simulink model "Punto_5"  (R2024b)
settings: Solver=VariableStepAuto  StartTime=0.0  StopTime=2  RelTol=1e-3
settings Model: Creator=Andres Felipe  LastModifiedBy=Andres Felipe

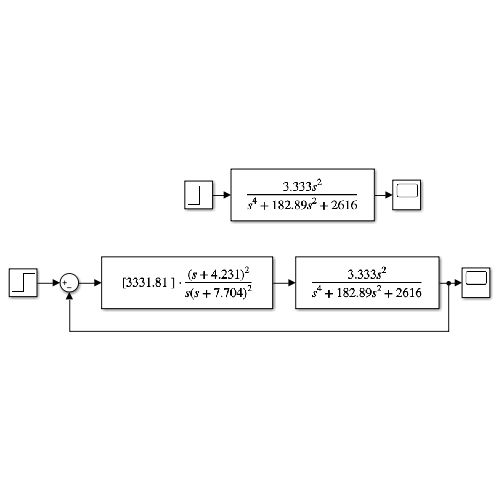
[thumbnail: Simulink's stored preview of the top-level diagram]
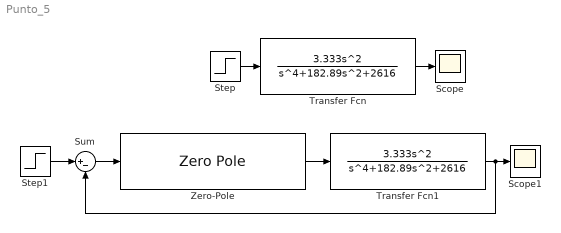
== system Punto_5 ==
  Scope : Scope
  Scope1 : Scope
  Step : Step  SampleTime=0
  Step1 : Step  SampleTime=0
  Sum : Sum  Inputs=|+-
  Transfer Fcn : TransferFcn  Numerator=[3.333 0 0]  Denominator=[1 0 182.89 0 2616]
  Transfer Fcn1 : TransferFcn  Numerator=[3.333 0 0]  Denominator=[1 0 182.89 0 2616]
  Zero-Pole : ZeroPole  Zeros=[-4.231 -4.231]  Poles=[0 -7.704 -7.704]  Gain=[3331.81]
  wires:
  Transfer Fcn/1 -> Scope/1
  Step/1 -> Transfer Fcn/1
  Transfer Fcn1/1 -> Sum/2, Scope1/1
  Step1/1 -> Sum/1
  Sum/1 -> Zero-Pole/1
  Zero-Pole/1 -> Transfer Fcn1/1
